simulink model "P45B_CCCV"  (R2025b)
settings: Solver=FixedStepDiscrete  StartTime=0.0  StopTime=stopTime  FixedStep=Ts  RelTol=1e-3
PostLoadFcn:
  | % Put the model folder on the MATLAB path, then load the parameters.
  | mdlDir = fileparts(get_param('P45B_CCCV','FileName'));
  | if ~isempty(mdlDir), addpath(mdlDir); end
  | clear mdlDir
  | if ~exist('Pack','var') || ~exist('Kp','var'), P45B('setup'); end
StopFcn:
  | P45B('plot');
values from neighbouring files (symbols this model uses):
  Ncells = evalin('base','Ncells')    [P45B.m]
  Np = evalin('base','Np')    [P45B.m]
  Ns = evalin('base','Ns')    [P45B.m]
undefined symbols (not defined in the file or in its folder): balCmd, balThreshold, battery_builder_rtmsupport, gcbh, Icharge, Iload, Iterm, Ki, Kp, Kt, loadN, loadNdelay, loadNon, SOC_minDischarge, SOC_resumeDischarge, Ts, V_recharge
libraries: simulink x6, nesl_utility x3, fl_lib x2, P45BPack_lib x1, BatteryCurrentManagement x1, BatteryBalancing x1
settings Model: Creator=nhamb  LastModifiedBy=nhamb
settings DataIOCC: SaveOutput=off  SaveTime=off  ReturnWorkspaceOutputs=off

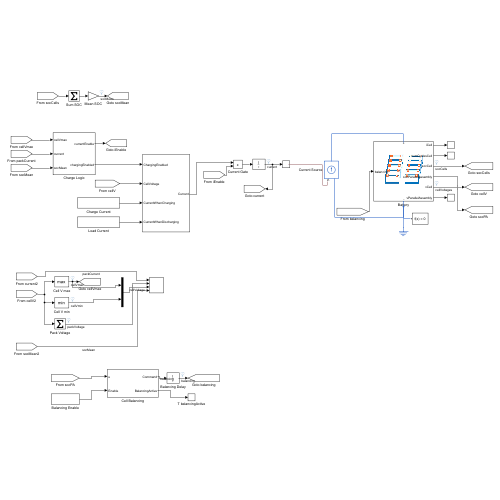
[thumbnail: Simulink's stored preview of the top-level diagram]
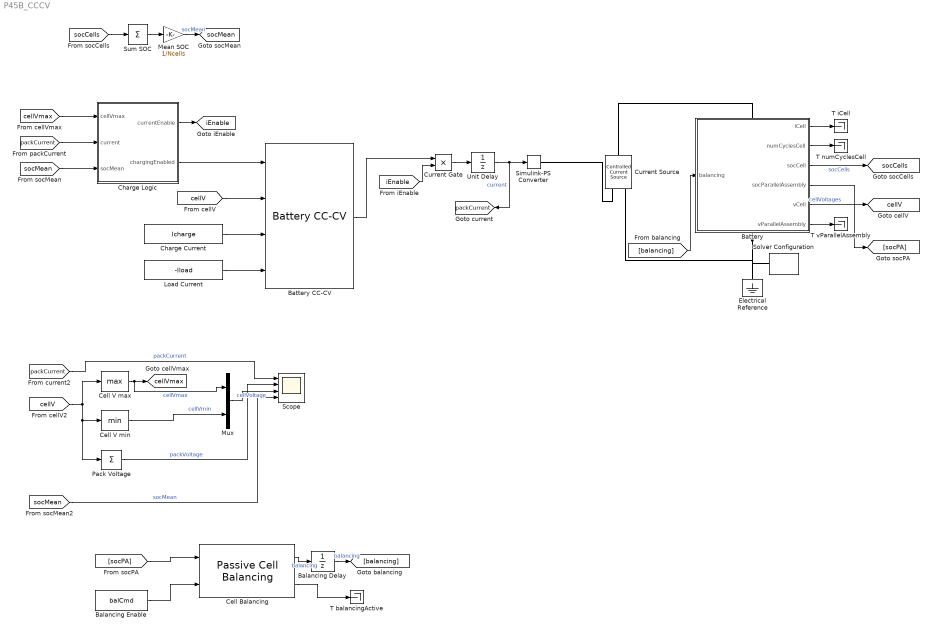
== system P45B_CCCV ==
  Balancing Delay : UnitDelay  SampleTime=Ts
  Balancing Enable : Constant  Value=balCmd
  Battery : Subsystem  LoadFcn=battery_builder_rtmsupport('loadfcn',gcbh);
      settings: CopyFcn=battery_builder_rtmsupport('copyfcn',gcbh);  PreCopyFcn=battery_builder_rtmsupport('precopyfcn',gcbh);  PreDeleteFcn=battery_builder_rtmsupport('predeletefcn',gcbh);  PortSchema="{\"entries\":[{\"content\":{\"sides\":[{\"content\":{\"connectorIds\":[\"LConn1\"]},\"type\":\"ConnectorPlacement.EquallySpacedRectSide\",\"uuid\":\"0463a81f-6a56-4adc-b9c0-eb6d89ee55b4\"},{\"content\":{\"connectorIds\":[\"RConn1\"],\"side\":\"RIGHT\"},\"type\":\"ConnectorPlacement.EquallySpacedRectSide\",\"uuid\":\"f93ae38f-9a35-4bc5-90d9-c500198b9c3c\"},{\"content\":{\"connectorIds\":[\"In1\"],\"side\":\"TOP\"},\"type\":\"ConnectorPlacement.EquallySpacedRectSide\",\"uuid\":\"e24de750-5e93-4785-b4b8-09f6c5f173af\"},{\"content\":{\"connectorIds\":[\"Out1\",\"Out2\",\"Out3\",\"Out4\",\"Out5\",\"Out6\"],\"side\":\"BOTTOM\"},\"type\":\"ConnectorPlacement.EquallySpacedRectSide\",\"uuid\":\"2e7e6c00-c53c-4615-9a66-6651fc426edd\"}]},\"type\":\"ConnectorPlacement.EquallySpacedConnector\",\"uuid\":\"e13c3efb-5cbd-456d-9e51-ec4146ffcf7f\"}],\"packageUris\":[\"http://schema.mathworks.com/mf0/Connector/R2020b\"],\"version\":\"1.0\"}"
      mask Display: image('$imagefile')
  Battery CC-CV : BatteryCurrentManagement/Battery CC-CV  MinMaxFlag=off  MaxCellVoltage=vMaxCell  Kp=Kp  Ki=Ki  Kaw=Kaw  Kt=Kt  Ts=Ts
  Cell Balancing : BatteryBalancing/Passive Cell Balancing  Threshold=balThreshold  HysteresisBand=balHysteresis  Td_on=balOnDelay  Td_off=balOffDelay  Ts=Ts  dataType=double
      settings: LibrarySourceBlock=batt_sl_lib/Cell Balancing/Passive Cell Balancing
  Cell V max : MinMax  Function=max
  Cell V min : MinMax
  Charge Current : Constant  Value=Icharge
  Charge Logic : Subsystem
  Current Gate : Product
  Current Source : fl_lib/Electrical/Electrical Sources/Controlled Current Source
  Electrical Reference : fl_lib/Electrical/Electrical Elements/Electrical Reference
  Load Current : Constant  Value=-Iload
  Mean SOC : Gain  Gain=1/Ncells
  Mux : Mux  Inputs=2
  Pack Voltage : Sum  Inputs=+
  Scope : Scope  NumInputPorts=4
      settings: ActiveDisplayYMinimum=-5.625  ActiveDisplayYMaximum=5.625
  Simulink-PS Converter : nesl_utility/Simulink-PS Converter  PhysicalDomain=network_engine_domain  SubClassName=ps_input  LeftPortType=input  RightPortType=output  PseudoPeriodic=off  Frequencies=[]  NoiseDistribution=none  NoiseParameters=[]  Unit=1  AffineConversion=off  FilteringAndDerivatives=provide  SimscapeFilterOrder=1  InputFilterTimeConstant=0.001  UdotUserProvided=0
  Solver Configuration : nesl_utility/Solver Configuration  PhysicalDomain=network_engine_domain  SubClassName=solver  LeftPortType=input  RightPortType=generic  Tones=[]  Harmonics=[]  SimulateNoise=off  Profile=off  UseLocalSampling=off  EnableSwitchedLinearOptims=on  FrequencyDomain=off  UseCCode=off  RelTol=0.001  AbsTol=0.001  MinStep=1e-09  ToWorkspace=off  RevertToSquareIcSolve=off  NumHomotopyIterations=100  PhasorMode=off  PhasorModeNumHarmonics=1  ConsistencySolver=NEWTON_XTOL_AFTER_FTOL  IndexReductionMethod=DerivativeReplacement  DoDC=off  ResidualTolerance=1e-09  ConsistencyTolSource=GLOBAL  ConsistencyAbsTol=0.001  ConsistencyRelTol=0.001  ConsistencyTolFactor=0.001  UseLocalSolver=on  LocalSolverChoice=NE_BACKWARD_EULER_ADVANCER  ResolveIndetEquations=on  FunctionEvalNumThread=1  LocalSolverSampleTime=Ts  DoFixedCost=on  MaxNonlinIter=3  MaxModeIter=2  ComputeImpulses=off  ImpulseIterations=2  LinearAlgebra=auto  LinearAlgebraNumThread=0  EquationFormulation=NE_TIME_EF  DelaysMemoryBudget=1024  AutomaticFiltering=on  FilteringTimeConstant=0.001  PartitionStorageMethod=AS_NEEDED  PartitionMemoryBudget=1024  PartitionMethod=ROBUST  MultibodyUseLocalSolver=off  MultibodyLocalSolverChoice=ODE1  MultibodyLocalSolverSampleTime=0.001
  Sum SOC : Sum  Inputs=+
  T balancingActive : Terminator
  T iCell : Terminator
  T numCyclesCell : Terminator
  T vParallelAssembly : Terminator
  Unit Delay : UnitDelay  SampleTime=Ts  HasFrameUpgradeWarning=on
  tag scope: cellV=global, cellVmax=global, iEnable=global, packCurrent=global, socCells=global, socMean=global
  wires:
  [socCells] -> Sum SOC/1
  Sum SOC/1 -> Mean SOC/1
  Mean SOC/1 -> [socMean]  "socMean"
  [cellVmax] -> Charge Logic/1(cellVmax)
  [packCurrent] -> Charge Logic/2(current)
  [socMean] -> Charge Logic/3(socMean)
  [cellV] -> Battery CC-CV/2
  Charge Current/1 -> Battery CC-CV/3
  Load Current/1 -> Battery CC-CV/4
  Unit Delay/1 -> [packCurrent], Simulink-PS Converter/1  "current"
  [cellV] -> Cell V min/1, Pack Voltage/1, Cell V max/1
  Cell V max/1 -> [cellVmax], Mux/1  "cellVmax"
  [packCurrent] -> Scope/1  "packCurrent"
  Pack Voltage/1 -> Scope/2  "packVoltage"
  Cell V min/1 -> Mux/2  "cellVmin"
  Mux/1 -> Scope/3  "cellVoltage"
  [socMean] -> Scope/4  "socMean"
  Charge Logic/1(currentEnable) -> [iEnable]
  Battery CC-CV/1 -> Current Gate/1
  [iEnable] -> Current Gate/2
  Current Gate/1 -> Unit Delay/1
  Charge Logic/2(chargingEnabled) -> Battery CC-CV/1
  Battery/1(iCell) -> T iCell/1
  Battery/2(numCyclesCell) -> T numCyclesCell/1
  Battery/3(socCell) -> [socCells]  "socCells"
  Battery/5(vCell) -> [cellV]  "cellVoltages"
  Battery/6(vParallelAssembly) -> T vParallelAssembly/1
  [socPA] -> Cell Balancing/1
  Balancing Enable/1 -> Cell Balancing/2
  Cell Balancing/2 -> T balancingActive/1
  [balancing] -> Battery/1(balancing)
  Cell Balancing/1 -> Balancing Delay/1  "balancing"
  Balancing Delay/1 -> [balancing]  "balancing"
  Battery/4(socParallelAssembly) -> [socPA]
  connections:
  Battery/LConn1 -- Current Source/LConn1
  Current Source/RConn2 -- Battery/RConn1 -- Electrical Reference/LConn1 -- Solver Configuration/RConn1
  Simulink-PS Converter/RConn1 -- Current Source/RConn1

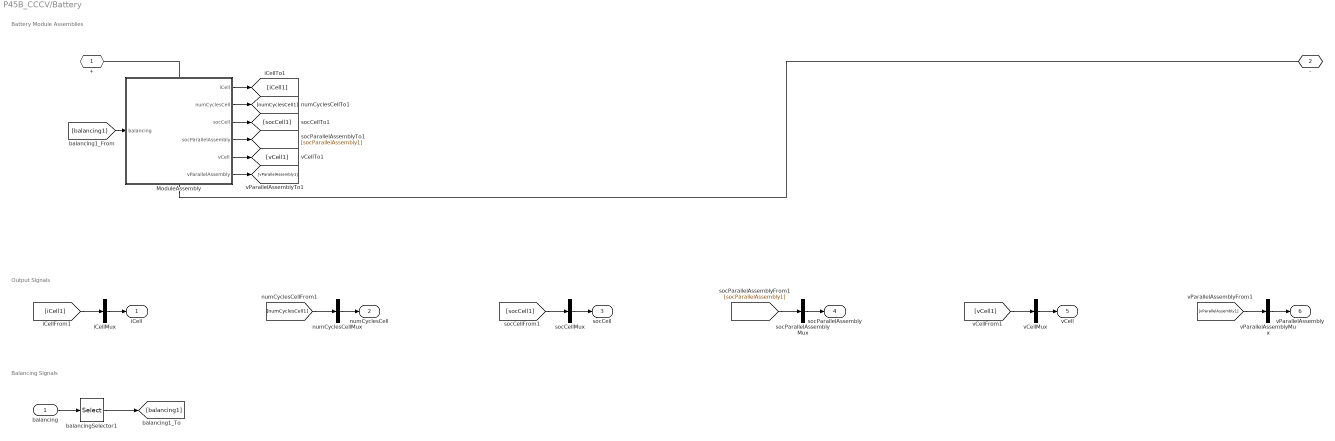
== system P45B_CCCV/Battery ==
  note: Battery Module Assemblies
  note: Output Signals
  note: Balancing Signals
  balancing : Inport  PortDimensions=Ns
  ModuleAssembly : Subsystem  LoadFcn=battery_builder_rtmsupport('loadfcn',gcbh);
      settings: CopyFcn=battery_builder_rtmsupport('copyfcn',gcbh);  PreCopyFcn=battery_builder_rtmsupport('precopyfcn',gcbh);  PreDeleteFcn=battery_builder_rtmsupport('predeletefcn',gcbh);  PortSchema="{\"entries\":[{\"content\":{\"sides\":[{\"content\":{\"connectorIds\":[\"LConn1\"]},\"type\":\"ConnectorPlacement.EquallySpacedRectSide\",\"uuid\":\"0463a81f-6a56-4adc-b9c0-eb6d89ee55b4\"},{\"content\":{\"connectorIds\":[\"RConn1\"],\"side\":\"RIGHT\"},\"type\":\"ConnectorPlacement.EquallySpacedRectSide\",\"uuid\":\"f93ae38f-9a35-4bc5-90d9-c500198b9c3c\"},{\"content\":{\"connectorIds\":[\"In1\"],\"side\":\"TOP\"},\"type\":\"ConnectorPlacement.EquallySpacedRectSide\",\"uuid\":\"e24de750-5e93-4785-b4b8-09f6c5f173af\"},{\"content\":{\"connectorIds\":[\"Out1\",\"Out2\",\"Out3\",\"Out4\",\"Out5\",\"Out6\"],\"side\":\"BOTTOM\"},\"type\":\"ConnectorPlacement.EquallySpacedRectSide\",\"uuid\":\"b6d424fb-e762-4d80-9247-db6b76e6c6f6\"}]},\"type\":\"ConnectorPlacement.EquallySpacedConnector\",\"uuid\":\"e13c3efb-5cbd-456d-9e51-ec4146ffcf7f\"}],\"packageUris\":[\"http://schema.mathworks.com/mf0/Connector/R2020b\"],\"version\":\"1.0\"}"
      mask Display: image('$imagefile')
  balancingSelector1 : Selector  InputPortWidth=Ns  IndexOptions=Index vector (dialog)  Indices=1:Ns  OutputSizes=1
  iCellMux : Mux  Inputs=1
  numCyclesCellMux : Mux  Inputs=1
  socCellMux : Mux  Inputs=1
  socParallelAssemblyMux : Mux  Inputs=1
  vCellMux : Mux  Inputs=1
  vParallelAssemblyMux : Mux  Inputs=1
  + : PMIOPort  Side=Left
  - : PMIOPort  Port=2  Side=Right
  iCell : Outport
  numCyclesCell : Outport  Port=2
  socCell : Outport  Port=3
  socParallelAssembly : Outport  Port=4
  vCell : Outport  Port=5
  vParallelAssembly : Outport  Port=6
  wires:
  ModuleAssembly/1(iCell) -> [iCell1]
  iCellMux/1 -> iCell/1
  [iCell1] -> iCellMux/1
  ModuleAssembly/2(numCyclesCell) -> [numCyclesCell1]
  numCyclesCellMux/1 -> numCyclesCell/1
  [numCyclesCell1] -> numCyclesCellMux/1
  ModuleAssembly/3(socCell) -> [socCell1]
  socCellMux/1 -> socCell/1
  [socCell1] -> socCellMux/1
  ModuleAssembly/4(socParallelAssembly) -> [socParallelAssembly1]
  socParallelAssemblyMux/1 -> socParallelAssembly/1
  [socParallelAssembly1] -> socParallelAssemblyMux/1
  ModuleAssembly/5(vCell) -> [vCell1]
  vCellMux/1 -> vCell/1
  [vCell1] -> vCellMux/1
  ModuleAssembly/6(vParallelAssembly) -> [vParallelAssembly1]
  vParallelAssemblyMux/1 -> vParallelAssembly/1
  [vParallelAssembly1] -> vParallelAssemblyMux/1
  [balancing1] -> ModuleAssembly/1(balancing)
  balancing/1 -> balancingSelector1/1
  balancingSelector1/1 -> [balancing1]
  connections:
  ModuleAssembly/LConn1 -- +/RConn1
  ModuleAssembly/RConn1 -- -/RConn1

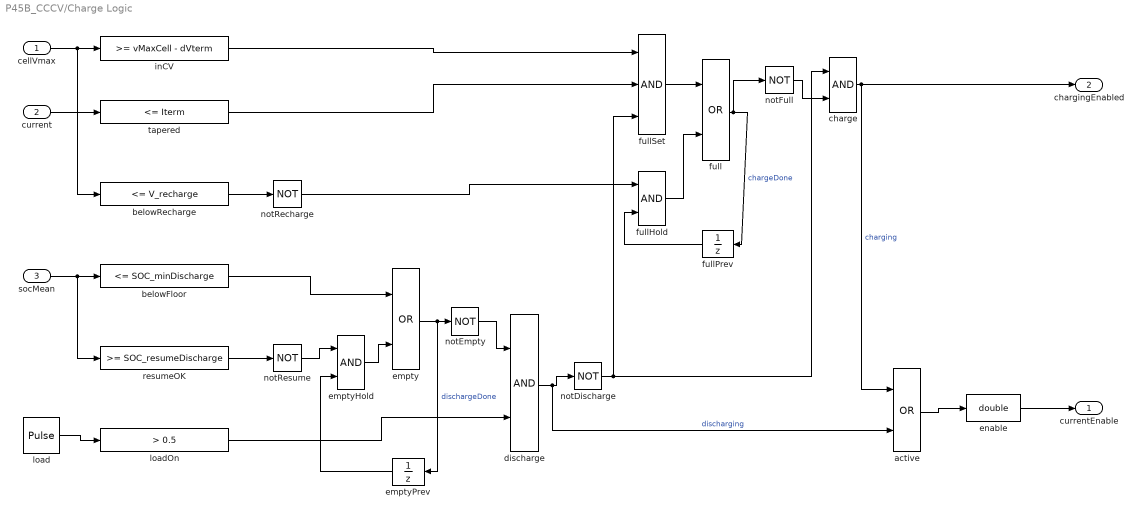
== system P45B_CCCV/Charge Logic ==
  cellVmax : Inport
  current : Inport  Port=2
  socMean : Inport  Port=3
  active : Logic  Operator=OR  AllPortsSameDT=off  OutDataTypeStr=boolean
  belowFloor : simulink/Logic and Bit Operations/Compare To Constant  relop=<=  const=SOC_minDischarge  OutDataTypeStr=boolean
  belowRecharge : simulink/Logic and Bit Operations/Compare To Constant  relop=<=  const=V_recharge  OutDataTypeStr=boolean
  charge : Logic  AllPortsSameDT=off  OutDataTypeStr=boolean
  discharge : Logic  AllPortsSameDT=off  OutDataTypeStr=boolean
  empty : Logic  Operator=OR  AllPortsSameDT=off  OutDataTypeStr=boolean
  emptyHold : Logic  AllPortsSameDT=off  OutDataTypeStr=boolean
  emptyPrev : UnitDelay  SampleTime=Ts  HasFrameUpgradeWarning=on
  enable : DataTypeConversion  OutDataTypeStr=double  SaturateOnIntegerOverflow=off  RndMeth=Floor
  full : Logic  Operator=OR  AllPortsSameDT=off  OutDataTypeStr=boolean
  fullHold : Logic  AllPortsSameDT=off  OutDataTypeStr=boolean
  fullPrev : UnitDelay  SampleTime=Ts  HasFrameUpgradeWarning=on
  fullSet : Logic  Inputs=3  AllPortsSameDT=off  OutDataTypeStr=boolean
  inCV : simulink/Logic and Bit Operations/Compare To Constant  relop=>=  const=vMaxCell - dVterm  OutDataTypeStr=boolean
  load : DiscretePulseGenerator  Period=loadN  PulseWidth=loadNon  PhaseDelay=loadNdelay  SampleTime=Ts
  loadOn : simulink/Logic and Bit Operations/Compare To Constant  relop=>  const=0.5  OutDataTypeStr=boolean
  notDischarge : Logic  Operator=NOT  Inputs=1  AllPortsSameDT=off  OutDataTypeStr=boolean
  notEmpty : Logic  Operator=NOT  Inputs=1  AllPortsSameDT=off  OutDataTypeStr=boolean
  notFull : Logic  Operator=NOT  Inputs=1  AllPortsSameDT=off  OutDataTypeStr=boolean
  notRecharge : Logic  Operator=NOT  Inputs=1  AllPortsSameDT=off  OutDataTypeStr=boolean
  notResume : Logic  Operator=NOT  Inputs=1  AllPortsSameDT=off  OutDataTypeStr=boolean
  resumeOK : simulink/Logic and Bit Operations/Compare To Constant  relop=>=  const=SOC_resumeDischarge  OutDataTypeStr=boolean
  tapered : simulink/Logic and Bit Operations/Compare To Constant  relop=<=  const=Iterm  OutDataTypeStr=boolean
  currentEnable : Outport
  chargingEnabled : Outport  Port=2
  wires:
  cellVmax/1 -> inCV/1, belowRecharge/1
  current/1 -> tapered/1
  socMean/1 -> belowFloor/1, resumeOK/1
  load/1 -> loadOn/1
  resumeOK/1 -> notResume/1
  emptyPrev/1 -> emptyHold/2
  notResume/1 -> emptyHold/1
  belowFloor/1 -> empty/1
  emptyHold/1 -> empty/2
  empty/1 -> emptyPrev/1, notEmpty/1  "dischargeDone"
  notEmpty/1 -> discharge/1
  loadOn/1 -> discharge/2
  discharge/1 -> active/2, notDischarge/1  "discharging"
  belowRecharge/1 -> notRecharge/1
  notRecharge/1 -> fullHold/1
  fullPrev/1 -> fullHold/2
  inCV/1 -> fullSet/1
  tapered/1 -> fullSet/2
  notDischarge/1 -> fullSet/3, charge/1
  fullSet/1 -> full/1
  fullHold/1 -> full/2
  full/1 -> fullPrev/1, notFull/1  "chargeDone"
  notFull/1 -> charge/2
  charge/1 -> active/1, chargingEnabled/1  "charging"
  active/1 -> enable/1
  enable/1 -> currentEnable/1

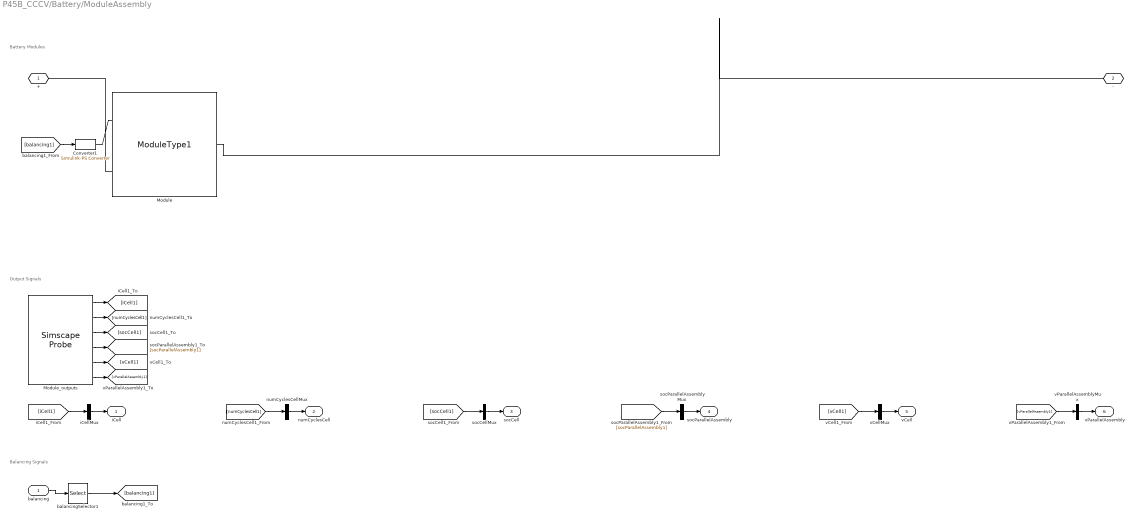
== system P45B_CCCV/Battery/ModuleAssembly ==
  note: Balancing Signals
  note: Output Signals
  note: Battery Modules
  balancing : Inport  PortDimensions=Ns
  Converter1 : nesl_utility/Simulink-PS Converter  PhysicalDomain=network_engine_domain  SubClassName=ps_input  LeftPortType=input  RightPortType=output  PseudoPeriodic=off  Frequencies=[]  NoiseDistribution=none  NoiseParameters=[]  Unit=1  AffineConversion=off  FilteringAndDerivatives=provide  SimscapeFilterOrder=1  InputFilterTimeConstant=0.001  UdotUserProvided=0
  Module : P45BPack_lib/Modules/ModuleType1  SOC_vecCell=Pack.SOC_vecCell  SOC_vecCellPercentDeviation=Pack.SOC_vecCellPercentDeviation  V0_vecCell=Pack.V0_vecCell V  V0_vecCellPercentDeviation=Pack.V0_vecCellPercentDeviation  V_rangeCell=Pack.V_rangeCell V  V_rangeCellPercentDeviation=Pack.V_rangeCellPercentDeviation  R0_vecCell=Pack.R0_vecCell Ohm  R0_vecCellPercentDeviation=Pack.R0_vecCellPercentDeviation  AHCell=Pack.AHCell A*hr  AHCellPercentDeviation=Pack.AHCellPercentDeviation  extrapolation_optionCell=simscape.enum.extrapolation.nearest  R1_vecCell=Pack.R1_vecCell Ohm  R1_vecCellPercentDeviation=Pack.R1_vecCellPercentDeviation  tau1_vecCell=Pack.tau1_vecCell s  tau1_vecCellPercentDeviation=Pack.tau1_vecCellPercentDeviation  CellBalancingClosedResistance=Pack.CellBalancingClosedResistance Ohm  CellBalancingOpenConductance=Pack.CellBalancingOpenConductance 1/Ohm  CellBalancingThreshold=Pack.CellBalancingThreshold  CellBalancingResistance=Pack.CellBalancingResistance Ohm  P=Np  S=Ns  iCell_specify=off  iCell_priority=None  iCell=repmat(0, 195, 1) A  iCell_nominal_specify=off  iCell_nominal_value=1  iCell_nominal_unit=A  vCell_specify=off  vCell_priority=None  vCell=repmat(0, 195, 1) V  vCell_nominal_specify=off  vCell_nominal_value=1  vCell_nominal_unit=V  socCell_specify=on  socCell_priority=High  socCell=SOC0Cell  socCell_nominal_specify=off  socCell_nominal_value=1  socCell_nominal_unit=1  numCyclesCell_specify=off  numCyclesCell_priority=High  numCyclesCell=repmat(0, 195, 1)  numCyclesCell_nominal_specify=off  numCyclesCell_nominal_value=1  numCyclesCell_nominal_unit=1  vParallelAssembly_specify=off  vParallelAssembly_priority=None  vParallelAssembly=repmat(0, 195, 1) V  vParallelAssembly_nominal_specify=off  vParallelAssembly_nominal_value=1  vParallelAssembly_nominal_unit=V  socParallelAssembly_specify=off  socParallelAssembly_priority=None  socParallelAssembly=repmat(1, 195, 1)  socParallelAssembly_nominal_specify=off  socParallelAssembly_nominal_value=1  socParallelAssembly_nominal_unit=1
      settings: InternalSimscapePortConfiguration="{\"Bottom\":[{\"id\":\"n\",\"label\":\"-\",\"type\":\"foundation.electrical.electrical\"}],\"Left\":[{\"id\":\"enableCellBalancing\",\"label\":\"CB\",\"type\":\"input\"}],\"Right\":[],\"Top\":[{\"id\":\"p\",\"label\":\"+\",\"type\":\"foundation.electrical.electrical\"}]}"
  Module_outputs : SimscapeProbe  BoundBlock=142  Variables="{\"iCell\":{\"Probing\":\"ON\"},\"numCyclesCell\":{\"Probing\":\"ON\"},\"socCell\":{\"Probing\":\"ON\"},\"socParallelAssembly\":{\"Probing\":\"ON\"},\"vCell\":{\"Probing\":\"ON\"},\"vParallelAssembly\":{\"Probing\":\"ON\"}}"
  balancingSelector1 : Selector  InputPortWidth=Ns  IndexOptions=Index vector (dialog)  Indices=1:Ns  OutputSizes=1
  iCellMux : Mux  Inputs=1
  numCyclesCellMux : Mux  Inputs=1
  socCellMux : Mux  Inputs=1
  socParallelAssemblyMux : Mux  Inputs=1
  vCellMux : Mux  Inputs=1
  vParallelAssemblyMux : Mux  Inputs=1
  + : PMIOPort  Side=Left
  - : PMIOPort  Port=2  Side=Right
  iCell : Outport
  numCyclesCell : Outport  Port=2
  socCell : Outport  Port=3
  socParallelAssembly : Outport  Port=4
  vCell : Outport  Port=5
  vParallelAssembly : Outport  Port=6
  wires:
  balancingSelector1/1 -> [balancing1]
  balancing/1 -> balancingSelector1/1
  [balancing1] -> Converter1/1
  [vParallelAssembly1] -> vParallelAssemblyMux/1
  vParallelAssemblyMux/1 -> vParallelAssembly/1
  Module_outputs/6 -> [vParallelAssembly1]
  [vCell1] -> vCellMux/1
  vCellMux/1 -> vCell/1
  Module_outputs/5 -> [vCell1]
  [socParallelAssembly1] -> socParallelAssemblyMux/1
  socParallelAssemblyMux/1 -> socParallelAssembly/1
  Module_outputs/4 -> [socParallelAssembly1]
  [socCell1] -> socCellMux/1
  socCellMux/1 -> socCell/1
  Module_outputs/3 -> [socCell1]
  [numCyclesCell1] -> numCyclesCellMux/1
  numCyclesCellMux/1 -> numCyclesCell/1
  Module_outputs/2 -> [numCyclesCell1]
  [iCell1] -> iCellMux/1
  iCellMux/1 -> iCell/1
  Module_outputs/1 -> [iCell1]
  connections:
  Converter1/RConn1 -- Module/LConn1
  Module/RConn1 -- -/RConn1
  Module/LConn2 -- +/RConn1
